simulink model "Exp6_DPCM"  (R2026a)
settings: Solver=VariableStepAuto  StopTime=1
libraries: simulink x1
settings Model: Creator=yatha  LastModifiedBy=yatha

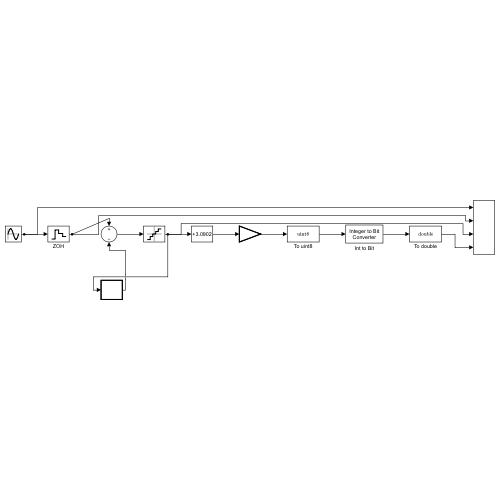
[thumbnail: Simulink's stored preview of the top-level diagram]
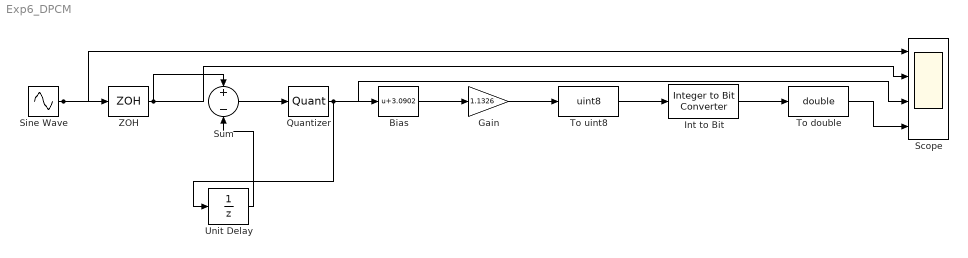
== system Exp6_DPCM ==
  Bias : Bias  Bias=3.0902  SaturateOnIntegerOverflow=off
  Gain : Gain  Gain=1.1326
  Int to Bit : simulink/Logic and Bit Operations/Integer to Bit Converter  nbits=3  signedInputValues=Unsigned  bitOrder=MSB first  outDtype=Inherit via internal rule
  Quantizer : Quantizer  QuantizationInterval=0.88291
  Scope : Scope  NumInputPorts=4
  Sine Wave : Sin  Amplitude=5  Frequency=12.5664  SampleTime=0
  Sum : Sum  Inputs=+-
  To double : DataTypeConversion  OutDataTypeStr=double  SaturateOnIntegerOverflow=off  RndMeth=Floor
  To uint8 : DataTypeConversion  OutDataTypeStr=uint8  SaturateOnIntegerOverflow=off  RndMeth=Floor
  Unit Delay : UnitDelay  SampleTime=0.05
  ZOH : ZeroOrderHold  SampleTime=0.05
  wires:
  Sine Wave/1 -> ZOH/1, Scope/1
  ZOH/1 -> Sum/1, Scope/2
  Sum/1 -> Quantizer/1
  Quantizer/1 -> Bias/1, Unit Delay/1, Scope/3
  Bias/1 -> Gain/1
  Gain/1 -> To uint8/1
  To uint8/1 -> Int to Bit/1
  Int to Bit/1 -> To double/1
  Unit Delay/1 -> Sum/2
  To double/1 -> Scope/4
